simulink model "Task_31"  (R2022b)
settings: Solver=VariableStepAuto  StartTime=0.0  StopTime=10.0  RelTol=1e-3
settings Model: Creator=Abanob_Sameh  LastModifiedBy=Abanob_Sameh

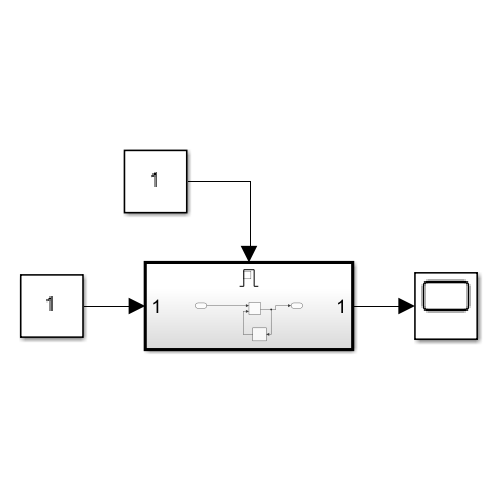
[thumbnail: Simulink's stored preview of the top-level diagram]
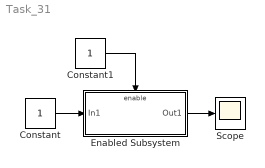
== system Task_31 ==
  Constant : Constant
  Constant1 : Constant
  Enabled Subsystem : Subsystem  TreatAsAtomicUnit=on
  Scope : Scope
  wires:
  Constant/1 -> Enabled Subsystem/1(In1)
  Enabled Subsystem/1(Out1) -> Scope/1
  Constant1/1 -> Enabled Subsystem/Enable

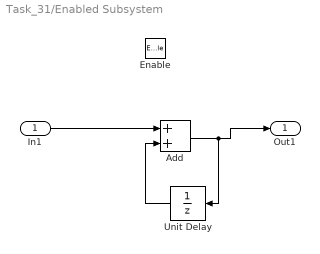
== system Task_31/Enabled Subsystem ==
  In1 : Inport
  Enable : EnablePort
  Add : Sum
  Unit Delay : UnitDelay  SampleTime=-1  HasFrameUpgradeWarning=on
  Out1 : Outport
  wires:
  In1/1 -> Add/1
  Unit Delay/1 -> Add/2
  Add/1 -> Unit Delay/1, Out1/1
